simulink model "gauss_seidel"  (R2021a)
settings: Solver=FixedStepDiscrete  StartTime=0.0  StopTime=10  FixedStep=1  RelTol=1e-3
libraries: dspinverses x1, simulink x1, dspmtrx3 x1
settings Model: Creator=manur  LastModifiedBy=manur

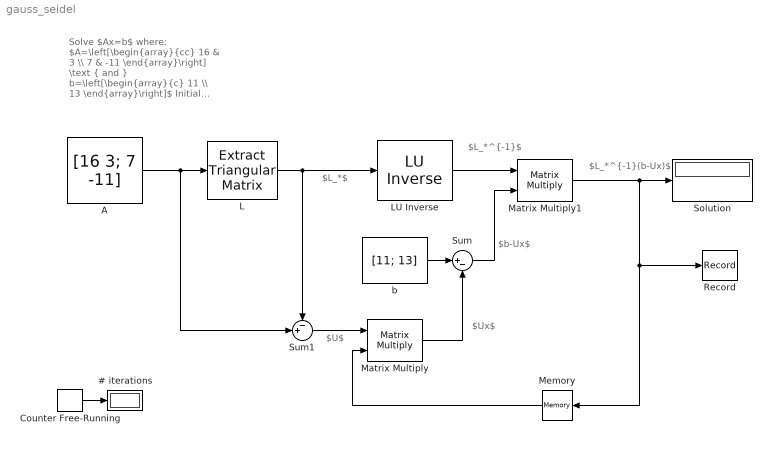
== system gauss_seidel ==
  note: Solve $Ax=b$ where:
      | $A=\left[\begin{array}{cc} 16 & 3 \\ 7 & -11 \end{array}\right] \text { and } b=\left[\begin{array}{c} 11 \\ 13 \end{array}\right]$
      | Initial guess is:
      | $x^{(0)}=\left[\begin{array}{l} 1.0 \\ 1.0 \end{array}\right]$
  note: $L_*$
  note: $L_*^{-1}$
  note: $U$
  note: $Ux$
  note: $b-Ux$
  note: $L_*^{-1}(b-Ux)$
  " LU Inverse" : dspinverses/ LU Inverse
  # iterations : Display
  A : Constant  Value=[16 3; 7 -11]
  Counter Free-Running : simulink/Sources/Counter Free-Running  NumBits=16  tsamp=-1
  L : dspmtrx3/Extract Triangular Matrix  fcn=Lower  SimulateUsing=Code generation
      settings: SourceProductBaseCode=DS
  Matrix Multiply : Product  Multiplication=Matrix(*)
  Matrix Multiply1 : Product  Multiplication=Matrix(*)
  Memory : Memory  InitialCondition=[1; 1]
  Record : Record  FileSettingsInternal="{\"entries\":[{\"content\":{\"excelSettings\":{\"content\":{},\"type\":\"Streamout.ExcelSettings\"}},\"type\":\"Streamout.FileSettingStorage\",\"uuid\":\"1f10d9fa-31e5-4a9f-8698-854757a7dd8a\"}],\"packageUris\":[\"http://schema.mathworks.com/mf0/streamout_blocks/R2020a\"],\"version\":\"1.0\"}"  Layout=[1 1]  SignalsInternal="{\"entries\":[{\"content\":{\"signals\":[{\"content\":{\"blockPath\":[\"gauss_seidel/Record\"],\"channel\":[],\"dimensions\":[2,1],\"domain\":\"gauss_seidel/record\",\"hasChildren\":true,\"lineColor\":\"#edb120\",\"plots\":[],\"port\":1,\"sid\":[],\"signalID\":62,\"signalName\":\"Matrix Multiply1\"},\"type\":\"RecordBlkView.Signal\",\"uuid\":\"c15fa9f7-8186-4076-943a-5077830479b2\"},{\"content\":{\"blockPath\":[\"gauss_seidel/Record\"],\"channel\":[1,1],\"dimensions\":[2,1],\"domain\":\"gauss_seidel/record\",\"lineColor\":\"#7e2f8e\",\"parentID\":62,\"plots\":[1],\"port\":1,\"sid\":[],\"signalID\":63,\"signalName\":\"Matrix Multiply1\"},\"type\":\"RecordBlkView.Signal\",\"uuid\":\"cae5b05a-129e-4ed3-9684-8e242d675fd3\"},{\"content\":{\"blockPath\":[\"gauss_seidel/Record\"],\"channel\":[2,1],\"dimensions\":[2,1],\"domain\":\"gauss_seidel/record\",\"lineColor\":\"#77ac30\",\"parentID\":62,\"plots\":[1],\"port\":1,\"sid\":[],\"signalID\":64,\"signalName\":\"Matrix Multiply1\"},\"type\":\"RecordBlkView.Signal\",\"uuid\":\"fc2e3dc6-e21d-4903-9130-368bd8c8cdf2\"}]},\"type\":\"RecordBlkView.InputSignals\",\"uuid\":\"1e0650b4-1e40-4d70-b3fa-fdad411eed5c\"}],\"packageUris\":[\"http://schema.mathworks.com/mf0/streamout_blocks/R2020a\"],\"version\":\"1.0\"}"  VisualizationBindings="{\"sparklinesplugin\":{\"info\":[{\"bindingParametersList\":[],\"subplotID\":1}]}}"
  Solution : Display
  Sum : Sum  Inputs=|+-
  Sum1 : Sum  Inputs=-+|
  b : Constant  Value=[11; 13]  VectorParams1D=off
  wires:
  Counter Free-Running/1 -> # iterations/1
  A/1 -> Sum1/2, L/1
  L/1 -> Sum1/1, " LU Inverse"/1
  b/1 -> Sum/1
  Matrix Multiply/1 -> Sum/2
  Sum/1 -> Matrix Multiply1/2
  " LU Inverse"/1 -> Matrix Multiply1/1
  Matrix Multiply1/1 -> Record/1, Memory/1, Solution/1
  Sum1/1 -> Matrix Multiply/1
  Memory/1 -> Matrix Multiply/2
